simulink model "Inner2_tmp"  (Simulink 8.3)
settings: Solver=FixedStepDiscrete  StartTime=0.0  StopTime=20.0  RelTol=1e-3
settings Model: Creator=scaife  LastModifiedBy=hbourbou  CovSFcnEnable=on  ExtModeAutoUpdateStatusClock=off
settings DataIOCC: SignalLoggingName=sigsOut
settings DebuggingCC: SaveWithParameterizedLinksMsg=none  SignalResolutionControl=TryResolveAllWithWarning  SolverPrmCheckMsg=none  MultiTaskDSMMsg=warning  MultiTaskCondExecSysMsg=none  FrameProcessingCompatibilityMsg=error  StateNameClashWarn=none
settings HardwareCC: TargetUnknown=on
settings SFSimCC: SimParseCustomCode=off

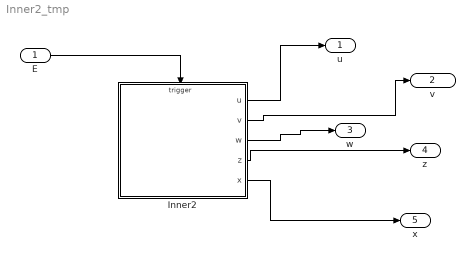
== system Inner2_tmp ==
  E : Inport
  Inner2 : Stateflow chart  TreatAsAtomicUnit=on
      settings: PermitHierarchicalResolution=ParametersOnly
  u : Outport
  v : Outport  Port=2
  w : Outport  Port=3
  z : Outport  Port=4
  x : Outport  Port=5
  wires:
  E/1 -> Inner2/Trigger
  Inner2/1(u) -> u/1
  Inner2/2(v) -> v/1
  Inner2/3(w) -> w/1
  Inner2/4(z) -> z/1
  Inner2/5(x) -> x/1

== stateflow chart Inner2 ==
  state A/
    en: u+=10000;
    ex: u+=100;
    du: u+=1;
    state A1/
      en: x+=10000;
      ex: x+=100;
      du: x+=1;
    state A2/
      en: v+=10000;
      ex: v+=100;
      du: v+=1;
    A -> A [order 1] : E[u%%3==0]{w++;}
    A -> A1 [order 2] : E[u%%3==1]
        | {x+=1000000;}
    A1 -> A : E[u%%3==2]
        | {z++;}
    (default) -> A2 : {v+=1000000;}
  (default) -> A
  data: u output int32; v output int32; w output int32; z output int32; x output int32
  events: E input EITHER_EDGE_EVENT
